simulink model "kundur_vsg"  (R2025b)
settings: Solver=ode23t  StartTime=0.0  StopTime=10.0  MaxStep=0.001  RelTol=1e-4
libraries: fl_lib x55, ee_lib x53, nesl_utility x17
(part 2 of 2)

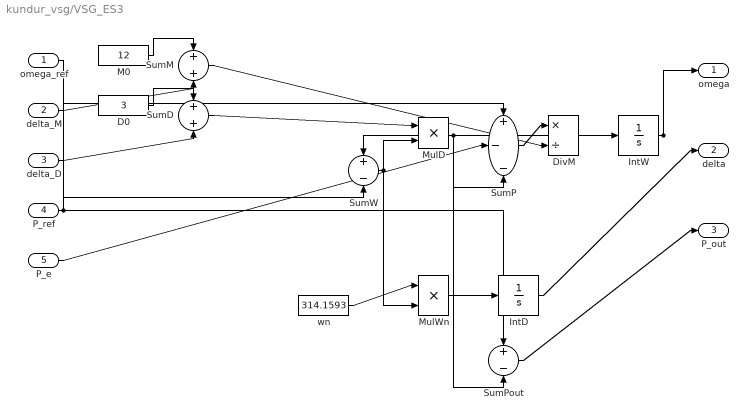
== system kundur_vsg/VSG_ES3 ==
  omega_ref : Inport
  delta_M : Inport  Port=2
  delta_D : Inport  Port=3
  P_ref : Inport  Port=4
  P_e : Inport  Port=5
  D0 : Constant  Value=3
  DivM : Product  Inputs=*/
  IntD : Integrator  InitialCondition=-0.095993
  IntW : Integrator  InitialCondition=1.0  LimitOutput=on  UpperSaturationLimit=1.1  LowerSaturationLimit=0.9
  M0 : Constant  Value=12
  MulD : Product  Inputs=**
  MulWn : Product  Inputs=**
  SumD : Sum
  SumM : Sum
  SumP : Sum  Inputs=+--
  SumPout : Sum  Inputs=+-
  SumW : Sum  Inputs=+-
  wn : Constant  Value=314.1593
  omega : Outport
  delta : Outport  Port=2
  P_out : Outport  Port=3
  wires:
  M0/1 -> SumM/1
  delta_M/1 -> SumM/2
  D0/1 -> SumD/1
  delta_D/1 -> SumD/2
  IntW/1 -> omega/1, SumW/1
  omega_ref/1 -> SumW/2
  SumD/1 -> MulD/1
  SumW/1 -> MulD/2, MulWn/2
  P_ref/1 -> SumP/1, SumPout/1
  P_e/1 -> SumP/2
  MulD/1 -> SumP/3, SumPout/2
  SumP/1 -> DivM/1
  SumM/1 -> DivM/2
  DivM/1 -> IntW/1
  wn/1 -> MulWn/1
  MulWn/1 -> IntD/1
  IntD/1 -> delta/1
  SumPout/1 -> P_out/1

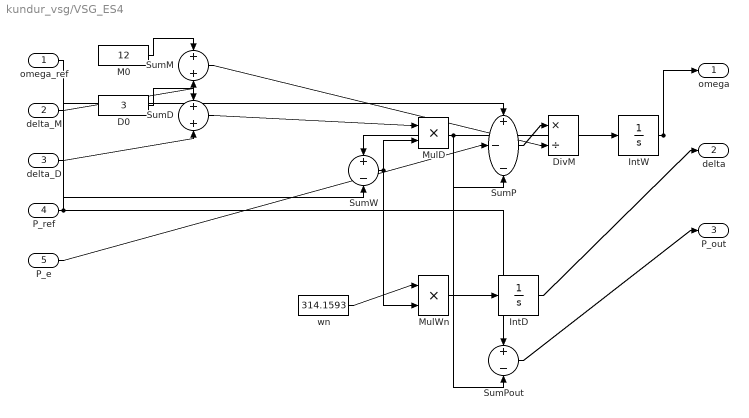
== system kundur_vsg/VSG_ES4 ==
  omega_ref : Inport
  delta_M : Inport  Port=2
  delta_D : Inport  Port=3
  P_ref : Inport  Port=4
  P_e : Inport  Port=5
  D0 : Constant  Value=3
  DivM : Product  Inputs=*/
  IntD : Integrator  InitialCondition=-0.061087
  IntW : Integrator  InitialCondition=1.0  LimitOutput=on  UpperSaturationLimit=1.1  LowerSaturationLimit=0.9
  M0 : Constant  Value=12
  MulD : Product  Inputs=**
  MulWn : Product  Inputs=**
  SumD : Sum
  SumM : Sum
  SumP : Sum  Inputs=+--
  SumPout : Sum  Inputs=+-
  SumW : Sum  Inputs=+-
  wn : Constant  Value=314.1593
  omega : Outport
  delta : Outport  Port=2
  P_out : Outport  Port=3
  wires:
  M0/1 -> SumM/1
  delta_M/1 -> SumM/2
  D0/1 -> SumD/1
  delta_D/1 -> SumD/2
  IntW/1 -> omega/1, SumW/1
  omega_ref/1 -> SumW/2
  SumD/1 -> MulD/1
  SumW/1 -> MulD/2, MulWn/2
  P_ref/1 -> SumP/1, SumPout/1
  P_e/1 -> SumP/2
  MulD/1 -> SumP/3, SumPout/2
  SumP/1 -> DivM/1
  SumM/1 -> DivM/2
  DivM/1 -> IntW/1
  wn/1 -> MulWn/1
  MulWn/1 -> IntD/1
  IntD/1 -> delta/1
  SumPout/1 -> P_out/1

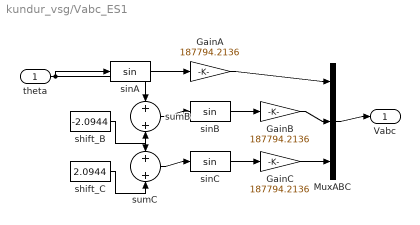
== system kundur_vsg/Vabc_ES1 ==
  theta : Inport
  GainA : Gain  Gain=187794.2136
  GainB : Gain  Gain=187794.2136
  GainC : Gain  Gain=187794.2136
  MuxABC : Mux  Inputs=3
  shift_B : Constant  Value=-2.0944
  shift_C : Constant  Value=2.0944
  sinA : Trigonometry
  sinB : Trigonometry
  sinC : Trigonometry
  sumB : Sum
  sumC : Sum
  Vabc : Outport
  wires:
  theta/1 -> sinA/1, sumB/1, sumC/1
  sinA/1 -> GainA/1
  shift_B/1 -> sumB/2
  sumB/1 -> sinB/1
  sinB/1 -> GainB/1
  shift_C/1 -> sumC/2
  sumC/1 -> sinC/1
  sinC/1 -> GainC/1
  GainA/1 -> MuxABC/1
  GainB/1 -> MuxABC/2
  GainC/1 -> MuxABC/3
  MuxABC/1 -> Vabc/1

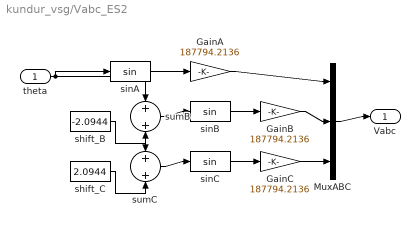
== system kundur_vsg/Vabc_ES2 ==
  theta : Inport
  GainA : Gain  Gain=187794.2136
  GainB : Gain  Gain=187794.2136
  GainC : Gain  Gain=187794.2136
  MuxABC : Mux  Inputs=3
  shift_B : Constant  Value=-2.0944
  shift_C : Constant  Value=2.0944
  sinA : Trigonometry
  sinB : Trigonometry
  sinC : Trigonometry
  sumB : Sum
  sumC : Sum
  Vabc : Outport
  wires:
  theta/1 -> sinA/1, sumB/1, sumC/1
  sinA/1 -> GainA/1
  shift_B/1 -> sumB/2
  sumB/1 -> sinB/1
  sinB/1 -> GainB/1
  shift_C/1 -> sumC/2
  sumC/1 -> sinC/1
  sinC/1 -> GainC/1
  GainA/1 -> MuxABC/1
  GainB/1 -> MuxABC/2
  GainC/1 -> MuxABC/3
  MuxABC/1 -> Vabc/1

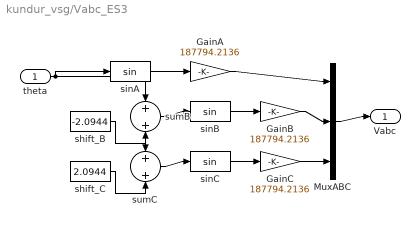
== system kundur_vsg/Vabc_ES3 ==
  theta : Inport
  GainA : Gain  Gain=187794.2136
  GainB : Gain  Gain=187794.2136
  GainC : Gain  Gain=187794.2136
  MuxABC : Mux  Inputs=3
  shift_B : Constant  Value=-2.0944
  shift_C : Constant  Value=2.0944
  sinA : Trigonometry
  sinB : Trigonometry
  sinC : Trigonometry
  sumB : Sum
  sumC : Sum
  Vabc : Outport
  wires:
  theta/1 -> sinA/1, sumB/1, sumC/1
  sinA/1 -> GainA/1
  shift_B/1 -> sumB/2
  sumB/1 -> sinB/1
  sinB/1 -> GainB/1
  shift_C/1 -> sumC/2
  sumC/1 -> sinC/1
  sinC/1 -> GainC/1
  GainA/1 -> MuxABC/1
  GainB/1 -> MuxABC/2
  GainC/1 -> MuxABC/3
  MuxABC/1 -> Vabc/1

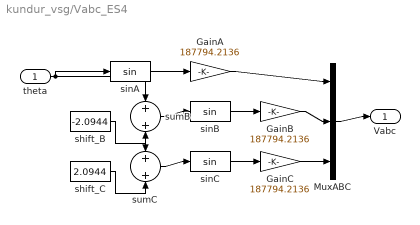
== system kundur_vsg/Vabc_ES4 ==
  theta : Inport
  GainA : Gain  Gain=187794.2136
  GainB : Gain  Gain=187794.2136
  GainC : Gain  Gain=187794.2136
  MuxABC : Mux  Inputs=3
  shift_B : Constant  Value=-2.0944
  shift_C : Constant  Value=2.0944
  sinA : Trigonometry
  sinB : Trigonometry
  sinC : Trigonometry
  sumB : Sum
  sumC : Sum
  Vabc : Outport
  wires:
  theta/1 -> sinA/1, sumB/1, sumC/1
  sinA/1 -> GainA/1
  shift_B/1 -> sumB/2
  sumB/1 -> sinB/1
  sinB/1 -> GainB/1
  shift_C/1 -> sumC/2
  sumC/1 -> sinC/1
  sinC/1 -> GainC/1
  GainA/1 -> MuxABC/1
  GainB/1 -> MuxABC/2
  GainC/1 -> MuxABC/3
  MuxABC/1 -> Vabc/1

== system kundur_vsg/Vabc_G1 ==
  theta : Inport
  GainA : Gain  Gain=193428.04
  GainB : Gain  Gain=193428.04
  GainC : Gain  Gain=193428.04
  MuxABC : Mux  Inputs=3
  shift_B : Constant  Value=-2.0944
  shift_C : Constant  Value=2.0944
  sinA : Trigonometry
  sinB : Trigonometry
  sinC : Trigonometry
  sumB : Sum
  sumC : Sum
  Vabc : Outport
  wires:
  theta/1 -> sinA/1, sumB/1, sumC/1
  sinA/1 -> GainA/1
  shift_B/1 -> sumB/2
  sumB/1 -> sinB/1
  sinB/1 -> GainB/1
  shift_C/1 -> sumC/2
  sumC/1 -> sinC/1
  sinC/1 -> GainC/1
  GainA/1 -> MuxABC/1
  GainB/1 -> MuxABC/2
  GainC/1 -> MuxABC/3
  MuxABC/1 -> Vabc/1

== system kundur_vsg/Vabc_G2 ==
  theta : Inport
  GainA : Gain  Gain=189672.1557
  GainB : Gain  Gain=189672.1557
  GainC : Gain  Gain=189672.1557
  MuxABC : Mux  Inputs=3
  shift_B : Constant  Value=-2.0944
  shift_C : Constant  Value=2.0944
  sinA : Trigonometry
  sinB : Trigonometry
  sinC : Trigonometry
  sumB : Sum
  sumC : Sum
  Vabc : Outport
  wires:
  theta/1 -> sinA/1, sumB/1, sumC/1
  sinA/1 -> GainA/1
  shift_B/1 -> sumB/2
  sumB/1 -> sinB/1
  sinB/1 -> GainB/1
  shift_C/1 -> sumC/2
  sumC/1 -> sinC/1
  sinC/1 -> GainC/1
  GainA/1 -> MuxABC/1
  GainB/1 -> MuxABC/2
  GainC/1 -> MuxABC/3
  MuxABC/1 -> Vabc/1

== system kundur_vsg/Vabc_G3 ==
  theta : Inport
  GainA : Gain  Gain=189672.1557
  GainB : Gain  Gain=189672.1557
  GainC : Gain  Gain=189672.1557
  MuxABC : Mux  Inputs=3
  shift_B : Constant  Value=-2.0944
  shift_C : Constant  Value=2.0944
  sinA : Trigonometry
  sinB : Trigonometry
  sinC : Trigonometry
  sumB : Sum
  sumC : Sum
  Vabc : Outport
  wires:
  theta/1 -> sinA/1, sumB/1, sumC/1
  sinA/1 -> GainA/1
  shift_B/1 -> sumB/2
  sumB/1 -> sinB/1
  sinB/1 -> GainB/1
  shift_C/1 -> sumC/2
  sumC/1 -> sinC/1
  sinC/1 -> GainC/1
  GainA/1 -> MuxABC/1
  GainB/1 -> MuxABC/2
  GainC/1 -> MuxABC/3
  MuxABC/1 -> Vabc/1
